simulink library "singleTetherNEqual2_cl"  (R2018b)
settings: Solver=VariableStepAuto  StartTime=0.0  StopTime=10.0  RelTol=1e-3
undefined symbols (not defined in the file or in its folder): gnd_station, ini_euler_ang, ini_Rcm_o, R11_g, R1n_cm, rotation_sequence, sim_param
libraries: tetherInternalForcesNEqual2_ul x1, tetherDragForceNEqual2_ul x1
settings Model: Creator=asiddiq2  LastModifiedBy=asiddiq2

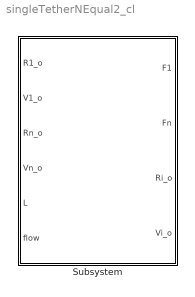
== system singleTetherNEqual2_cl ==
  Subsystem : Subsystem  mask{N=sim_param.N, dia_t=sim_param.tether_param.tether_diameter(1), E=sim_param.tether_param.tether_youngs, rho_tether=sim_param.tether_param.tether_density+ sim_param.env_param.density, Cd=sim_param.tether_param.CD_cylinder, zeta=sim_param.tether_param.damping_ratio, rho=sim_param.env_param.density, g=sim_param.env_param.grav, mass=sim_param.geom_param.mass, ini_Rn_o=ini_Rcm_o + rotation_sequence(ini_euler_ang)*R1n_cm, ini_R1_o=gnd_station + R11_g}
      mask prompts: N "Number of nodes (N>=2)"; dia_t "Tether diameter (m)"; E "Tether youngs modulus (N/m^2)"; rho_tether "Tether density (kg/m^3)"; Cd "Tether drag coefficient"; zeta "Damping ratio"; rho "Fluid density"; g "Gravitational acceleration"; mass "Vehicle mass"; ini_Rn_o "Initial vehicle attachment position vector"; ini_R1_o "Initial ground attachment position vector"
      mask init:
      | singleTether_init
      mask DialogControl Container2 Prompt: Tether properties

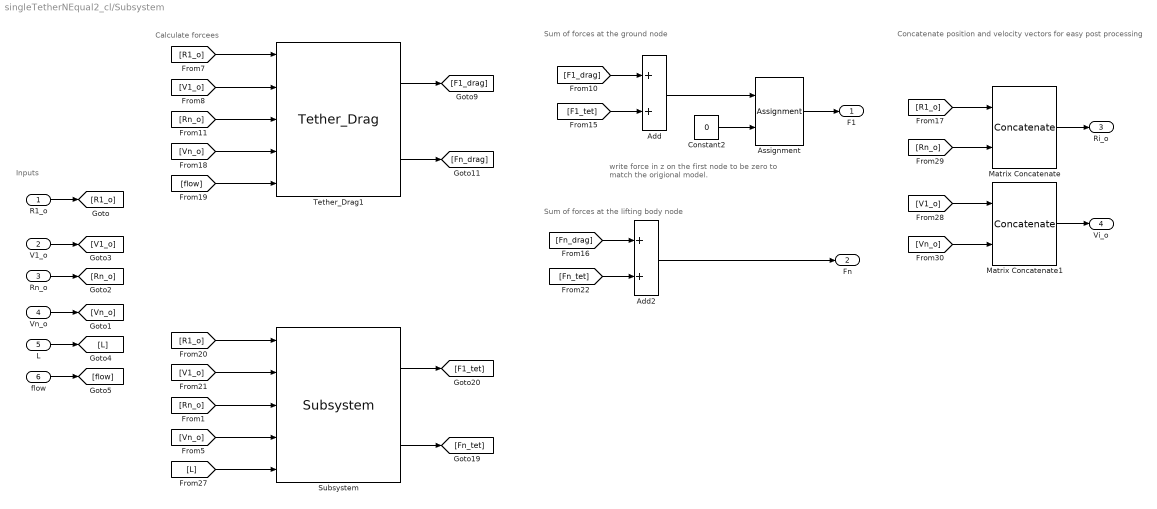
== system singleTetherNEqual2_cl/Subsystem ==
  note: Concatenate position and velocity vectors for easy
      | post processing
  note: Calculate forcees
  note: Sum of forces at the lifting body node
  note: Sum of forces at the ground node
  note: write force in z on the first node to be zero
      | to match the origional model.
  note: Inputs
  R1_o : Inport
  V1_o : Inport  Port=2
  Rn_o : Inport  Port=3
  Vn_o : Inport  Port=4
  L : Inport  Port=5
  flow : Inport  Port=6
  Add : Sum
  Add2 : Sum
  Assignment : Assignment  NumberOfDimensions=2  DiagnosticForDimensions=Warning  IndexOptions=Index vector (dialog),Index vector (dialog)  Indices=3,1  OutputSizes=1,1
  Constant2 : Constant  Value=0
  Matrix Concatenate : Concatenate  Mode=Multidimensional array  ConcatenateDimension=2
  Matrix Concatenate1 : Concatenate  Mode=Multidimensional array  ConcatenateDimension=2
  Subsystem : tetherInternalForcesNEqual2_ul/Subsystem  N=N  E=E  dia_t=dia_t  mass=mass  zeta=zeta
  Tether_Drag1 : tetherDragForceNEqual2_ul/Tether_Drag  Cd=Cd  rho_fluid=rho_fluid  dia_t=dia_t
  F1 : Outport
  Fn : Outport  Port=2
  Ri_o : Outport  Port=3
  Vi_o : Outport  Port=4
  wires:
  R1_o/1 -> [R1_o]
  V1_o/1 -> [V1_o]
  Rn_o/1 -> [Rn_o]
  Vn_o/1 -> [Vn_o]
  L/1 -> [L]
  flow/1 -> [flow]
  [F1_drag] -> Add/1
  [F1_tet] -> Add/2
  Assignment/1 -> F1/1
  Add/1 -> Assignment/1
  Constant2/1 -> Assignment/2
  Tether_Drag1/1 -> [F1_drag]
  Tether_Drag1/2 -> [Fn_drag]
  Subsystem/2 -> [Fn_tet]
  Subsystem/1 -> [F1_tet]
  [Fn_drag] -> Add2/1
  [Fn_tet] -> Add2/2
  Add2/1 -> Fn/1
  [R1_o] -> Tether_Drag1/1
  [V1_o] -> Tether_Drag1/2
  [Rn_o] -> Tether_Drag1/3
  [Vn_o] -> Tether_Drag1/4
  [flow] -> Tether_Drag1/5
  [Rn_o] -> Matrix Concatenate/2
  [R1_o] -> Matrix Concatenate/1
  Matrix Concatenate/1 -> Ri_o/1
  [V1_o] -> Matrix Concatenate1/1
  Matrix Concatenate1/1 -> Vi_o/1
  [Vn_o] -> Matrix Concatenate1/2
  [Vn_o] -> Subsystem/4
  [Rn_o] -> Subsystem/3
  [V1_o] -> Subsystem/2
  [R1_o] -> Subsystem/1
  [L] -> Subsystem/5
